simulink model "sliding_control"  (R2017a)
settings: Solver=FixedStepAuto  StartTime=0.0  StopTime=11  FixedStep=0.01  RelTol=1e-3
values from neighbouring files (symbols this model uses):
  a = 1    [sliding.m]
  eta = 2    [sliding.m]
  lambda = 1    [sliding.m]
  x1_0 = 3    [sliding.m]
  x2_0 = 0    [sliding.m]
undefined symbols (not defined in the file or in its folder): magnitude
settings Model: Creator=dell  LastModifiedBy=dell

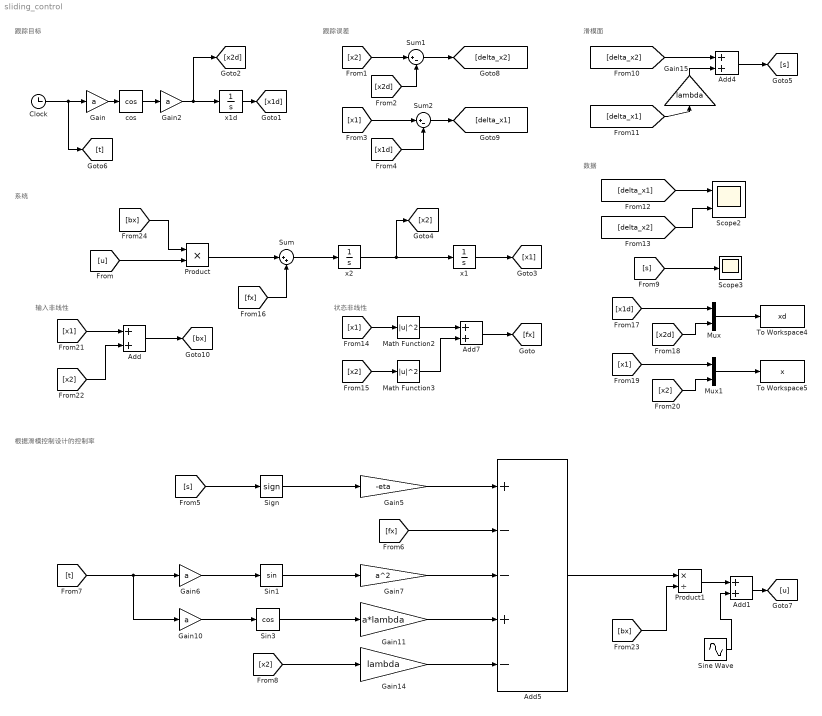
== system sliding_control ==
  note: 跟踪目标
  note: 滑模面
  note: 跟踪误差
  note: 输入非线性
  note: 根据滑模控制设计的控制率
  note: 系统
  note: 数据
  note: 状态非线性
  Add{,1,4,7} (4 alike) : Sum
  Add5 : Sum  Inputs=+--+-
  Clock : Clock
  Gain{,2,6,10} (4 alike) : Gain  Gain=a
  Gain11 : Gain  Gain=a*lambda
  Gain14 : Gain  Gain=lambda
  Gain15 : Gain  Gain=lambda
  Gain5 : Gain  Gain=-eta
  Gain7 : Gain  Gain=a^2
  Math Function2 : Math  Operator=magnitude^2  SaturateOnIntegerOverflow=on
  Math Function3 : Math  Operator=magnitude^2  SaturateOnIntegerOverflow=on
  Mux : Mux  Inputs=2
  Mux1 : Mux  Inputs=2
  Product : Product
  Product1 : Product  Inputs=*/
  Scope2 : Scope  NumInputPorts=2
  Scope3 : Scope
  Sign : Signum  ZeroCross=off
  Sin1 : Trigonometry
  Sin3 : Trigonometry  Operator=cos
  Sine Wave : Sin  Amplitude=0.1  Bias=0.02  Frequency=20  Phase=2  SampleTime=0
  Sum : Sum  Inputs=|++
  Sum1 : Sum  Inputs=|+-
  Sum2 : Sum  Inputs=|+-
  To Workspace4 : ToWorkspace  VariableName=xd  SampleTime=-1
  To Workspace5 : ToWorkspace  VariableName=x  SampleTime=-1
  cos : Trigonometry  Operator=cos
  x1 : Integrator  InitialCondition=x1_0
  x1d : Integrator
  x2 : Integrator  InitialCondition=x2_0
  wires:
  Mux1/1 -> To Workspace5/1
  Math Function2/1 -> Add7/1
  [delta_x1] -> Gain15/1
  [x2] -> Math Function3/1
  [fx] -> Sum/2
  Add7/1 -> [fx]
  Add/1 -> [bx]
  Math Function3/1 -> Add7/2
  Clock/1 -> [t], Gain/1
  [x1] -> Math Function2/1
  cos/1 -> Gain2/1
  Gain14/1 -> Add5/5
  [s] -> Scope3/1
  [x1] -> Mux1/1
  Gain11/1 -> Add5/4
  Product/1 -> Sum/1
  [x2d] -> Mux/2
  Add5/1 -> Product1/1
  Sum1/1 -> [delta_x2]
  Gain6/1 -> Sin1/1
  [delta_x1] -> Scope2/1
  [x2] -> Gain14/1
  Product1/1 -> Add1/1
  [x1d] -> Mux/1
  x2/1 -> [x2], x1/1
  Sign/1 -> Gain5/1
  [t] -> Gain6/1, Gain10/1
  Sin3/1 -> Gain11/1
  Gain7/1 -> Add5/3
  Mux/1 -> To Workspace4/1
  [x2d] -> Sum1/2
  [delta_x2] -> Add4/1
  [bx] -> Product1/2
  [x1] -> Sum2/1
  Gain2/1 -> x1d/1, [x2d]
  [x2] -> Sum1/1
  Gain5/1 -> Add5/1
  [s] -> Sign/1
  x1d/1 -> [x1d]
  Add4/1 -> [s]
  Sum2/1 -> [delta_x1]
  [x1d] -> Sum2/2
  [x2] -> Mux1/2
  [u] -> Product/2
  Sin1/1 -> Gain7/1
  Sum/1 -> x2/1
  [fx] -> Add5/2
  Gain10/1 -> Sin3/1
  [delta_x2] -> Scope2/2
  x1/1 -> [x1]
  Gain15/1 -> Add4/2
  Gain/1 -> cos/1
  [x1] -> Add/1
  [x2] -> Add/2
  [bx] -> Product/1
  Add1/1 -> [u]
  Sine Wave/1 -> Add1/2
